simulink model "SIL_Autopilot_Vasarhelyi"  (R2020b)
settings: Solver=FixedStepAuto  StartTime=0  StopTime=T  FixedStep=0.01  RelTol=1e-3  EnableMultiTasking=on
model workspace (MAT data in the model file):
  SL_ROS_VariableLengthArrays_MaxSizes : object (value not decoded)
undefined symbols (not defined in the file): Altitude_ref, DiscIntNeverNeededParam, Elevators, p_swarm, Propeller, RightAileron, RightFlap, Rudder
libraries: robotlib x20, simulink x15
(part 5 of 5)

== matlab function SIL_Autopilot_Vasarhelyi/Cessna 1/Local Flocking Algorithm/Gerador de Waypoints/Próximo Waypoint ==
  data: X_ref output; wp1_X input; wp1_Y input; wp2_X input; wp2_Y input; wp3_X input; wp3_Y input; wp4_X input; wp4_Y input; Y_med input; X_med input; Y_ref output; Estado output; Estado input
function [X_ref, Y_ref, Estado] = trajetoria(wp1_X, wp1_Y, wp2_X, wp2_Y,wp3_X, wp3_Y,wp4_X, wp4_Y, Y_med, X_med, Estado)

% Especifica o tamanho do raio.
R = 500;

switch (Estado)
    case 0 %seta o primeiro way point
        % WAY POINT 1
        X_ref = wp1_X;
        Y_ref = wp1_Y;
        %analisa se a aeronave atingiu o WAYPOINT
        if ( sqrt( (wp1_X - X_med)^2 +(wp1_Y - Y_med)^2) < R  )
         Estado = 1; %se sim: passa para o proximo WAYPOINT
        else
         Estado = 0;%se não: continua no mesmo WAYPONT
        end
    case 1
        % WAY POINT 2
        X_ref = wp2_X;
        Y_ref = wp2_Y;
        %analisa se a aeronave atingiu o WAYPOINT
        if ( sqrt((wp2_X - X_med)^2 +(wp2_Y - Y_med)^2) < R )
            Estado = 2;%se sim: passa para o proximo WAYPOINT
        else 
            Estado = 1;%se não: continua no mesmo WAYPONT
        end
    case 2
        % WAY POINT 3
        X_ref = wp3_X;
        Y_ref = wp3_Y;
        %analisa se a aeronave atingiu o WAYPOINT
        if ( sqrt( (wp3_X - X_med)^2 + (wp3_Y - Y_med)^2 ) < R )
            Estado = 3;%se sim: passa para o proximo WAYPOINT
        else 
            Estado = 2;%se não: continua no mesmo WAYPONT
        end
    case 3
        % WAY POINT 3
        X_ref = wp4_X;
        Y_ref = wp4_Y;
        %analisa se a aeronave atingiu o WAYPOINT
        if (sqrt( (wp4_X - X_med)^2 + (wp4_Y - Y_med)^2 )<R )
            Estado = 0;%se sim: passa para o proximo WAYPOINT
        else 
            Estado = 3;%se não: continua no mesmo WAYPONT
        end

    otherwise
        % seta o primeiro o waypoint
        X_ref = wp1_X;
        Y_ref = wp1_Y;
        Estado = 0;
end

end
